simulink model "missile_simulator"  (R2022b)
settings: Solver=VariableStepAuto  StartTime=0.0  StopTime=10  RelTol=1e-3
libraries: vrlib x9
settings Model: Creator=백창인  LastModifiedBy=snow

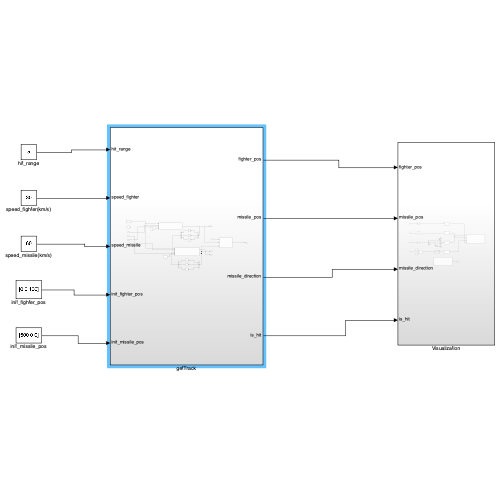
[thumbnail: Simulink's stored preview of the top-level diagram]
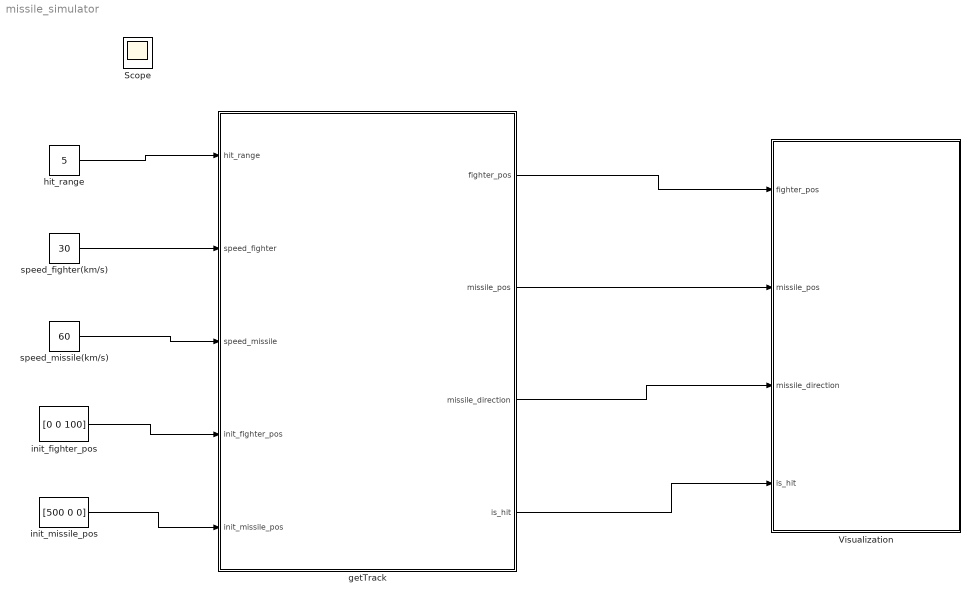
== system missile_simulator ==
  Visualization : Subsystem
  getTrack : Subsystem
  hit_range : Constant  Value=5
  init_fighter_pos : Constant  Value=[0 0 100]
  init_missile_pos : Constant  Value=[500 0 0]
  speed_fighter(km/s) : Constant  Value=30
  speed_missile(km/s) : Constant  Value=60
  Scope : Scope
  wires:
  hit_range/1 -> getTrack/1(hit_range)
  speed_fighter(km/s)/1 -> getTrack/2(speed_fighter)
  speed_missile(km/s)/1 -> getTrack/3(speed_missile)
  init_fighter_pos/1 -> getTrack/4(init_fighter_pos)
  init_missile_pos/1 -> getTrack/5(init_missile_pos)
  getTrack/3(missile_direction) -> Visualization/3(missile_direction)
  getTrack/2(missile_pos) -> Visualization/2(missile_pos)
  getTrack/1(fighter_pos) -> Visualization/1(fighter_pos)
  getTrack/4(is_hit) -> Visualization/4(is_hit)

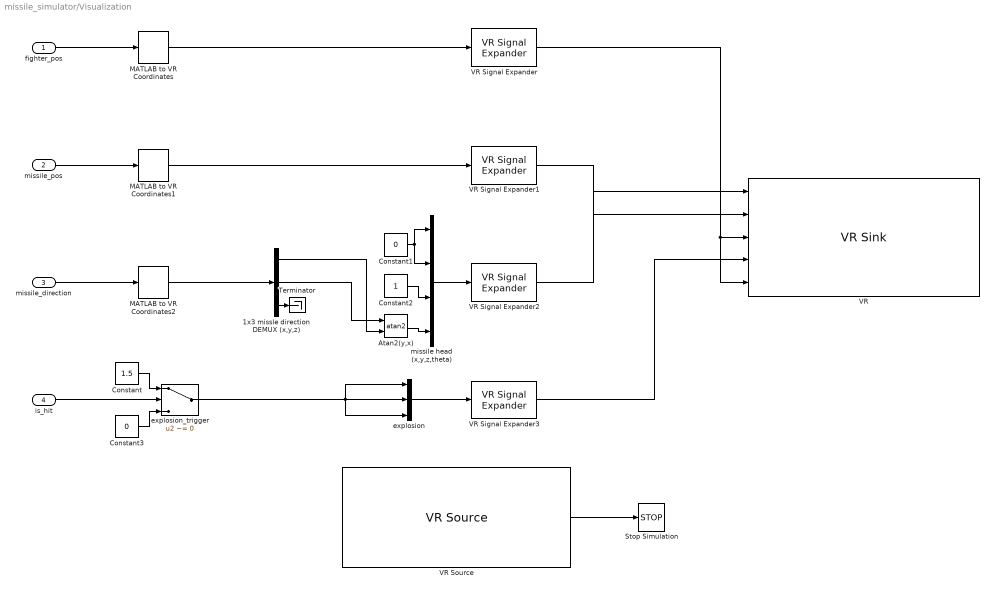
== system missile_simulator/Visualization ==
  fighter_pos : Inport
  missile_pos : Inport  Port=2
  missile_direction : Inport  Port=3
  is_hit : Inport  Port=4
  1x3 missle direction DEMUX (x,y,z) : Demux  Outputs=3
  Atan2(y,x) : Trigonometry  Operator=atan2
  Constant : Constant  Value=1.5
  Constant1 : Constant  Value=0
  Constant2 : Constant
  Constant3 : Constant  Value=0
  MATLAB to VR Coordinates : vrlib/Utilities/MATLAB to VR Coordinates
  MATLAB to VR Coordinates1 : vrlib/Utilities/MATLAB to VR Coordinates
  MATLAB to VR Coordinates2 : vrlib/Utilities/MATLAB to VR Coordinates
  Stop Simulation : Stop
  Terminator : Terminator
  VR : vrlib/VR Sink  InstantiateOnLoad=on  SampleTime=0.01  ViewEnable=on  RemoteChange=off  RemoteView=off  FieldsWritten=missile.rotation.4.1.1.double#missile.translation.3.1.1.double#Fighter.translation.3.1.1.double#explosion.scale.3.1.1.double#explosion.translation.3.1.1.double  WorldFileName=display.x3d  AutoView=on  VideoDimensions=[]  AllowVariableSize=off
  VR Signal Expander : vrlib/VR Signal Expander  outwidth=3  outidx=[1 2 3]
  VR Signal Expander1 : vrlib/VR Signal Expander  outwidth=3  outidx=[1 2 3]
  VR Signal Expander2 : vrlib/VR Signal Expander  outwidth=4  outidx=[1 2 3 4]
  VR Signal Expander3 : vrlib/VR Signal Expander  outwidth=3  outidx=[1 2 3]
  VR Source : vrlib/VR Source  InstantiateOnLoad=on  SampleTime=0.1  ViewEnable=on  RemoteChange=off  RemoteView=off  FieldsRead=explosion.scale.1.3.1.double  WorldFileName=display.x3d  AutoView=off  VideoDimensions=[]  AllowVariableSize=off
  explosion : Mux  Inputs=3
  explosion_trigger : Switch  Criteria=u2 ~= 0  SaturateOnIntegerOverflow=off  InputSameDT=off
  missile head (x,y,z,theta) : Mux
  wires:
  MATLAB to VR Coordinates/1 -> VR Signal Expander/1
  fighter_pos/1 -> MATLAB to VR Coordinates/1
  missile_pos/1 -> MATLAB to VR Coordinates1/1
  MATLAB to VR Coordinates1/1 -> VR Signal Expander1/1
  Constant2/1 -> missile head (x,y,z,theta)/3
  1x3 missle direction DEMUX (x,y,z)/1 -> Atan2(y,x)/2
  1x3 missle direction DEMUX (x,y,z)/2 -> Atan2(y,x)/1
  missile head (x,y,z,theta)/1 -> VR Signal Expander2/1
  Constant1/1 -> missile head (x,y,z,theta)/1, missile head (x,y,z,theta)/2
  Atan2(y,x)/1 -> missile head (x,y,z,theta)/4
  MATLAB to VR Coordinates2/1 -> 1x3 missle direction DEMUX (x,y,z)/1
  missile_direction/1 -> MATLAB to VR Coordinates2/1
  explosion/1 -> VR Signal Expander3/1
  explosion_trigger/1 -> explosion/1, explosion/3, explosion/2
  is_hit/1 -> explosion_trigger/2
  Constant3/1 -> explosion_trigger/3
  Constant/1 -> explosion_trigger/1
  1x3 missle direction DEMUX (x,y,z)/3 -> Terminator/1
  VR Signal Expander2/1 -> VR/1
  VR Signal Expander1/1 -> VR/2
  VR Signal Expander/1 -> VR/3, VR/5
  VR Signal Expander3/1 -> VR/4
  VR Source/1 -> Stop Simulation/1

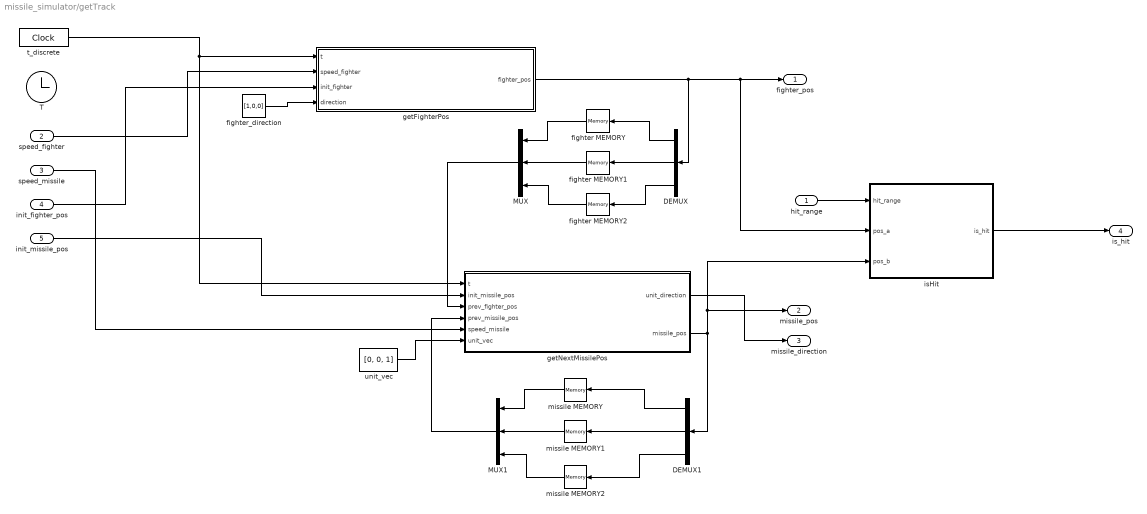
== system missile_simulator/getTrack ==
  hit_range : Inport
  speed_fighter : Inport  Port=2
  speed_missile : Inport  Port=3
  init_fighter_pos : Inport  Port=4
  init_missile_pos : Inport  Port=5
  DEMUX : Demux  Outputs=3
  DEMUX1 : Demux  Outputs=3
  MUX : Mux  Inputs=3
  MUX1 : Mux  Inputs=3
  T : Clock
  fighter MEMORY : Memory  InheritSampleTime=on
  fighter MEMORY1 : Memory  InheritSampleTime=on
  fighter MEMORY2 : Memory  InheritSampleTime=on
  fighter_direction : Constant  Value=[1,0,0]
  getFighterPos : MATLAB Function  TreatAsAtomicUnit=on
  getNextMissilePos : MATLAB Function  TreatAsAtomicUnit=on
  isHit : MATLAB Function  TreatAsAtomicUnit=on
  missile MEMORY : Memory  InheritSampleTime=on
  missile MEMORY1 : Memory  InheritSampleTime=on
  missile MEMORY2 : Memory  InheritSampleTime=on
  t_discrete : DigitalClock  SampleTime=0.001
  unit_vec : Constant  Value=[0, 0, 1]
  fighter_pos : Outport
  missile_pos : Outport  Port=2
  missile_direction : Outport  Port=3
  is_hit : Outport  Port=4
  wires:
  t_discrete/1 -> getNextMissilePos/1(t), getFighterPos/1(t)
  getFighterPos/1(fighter_pos) -> DEMUX/1, isHit/2(pos_a), fighter_pos/1
  speed_fighter/1 -> getFighterPos/2(speed_fighter)
  init_fighter_pos/1 -> getFighterPos/3(init_fighter)
  fighter_direction/1 -> getFighterPos/4(direction)
  getNextMissilePos/2(missile_pos) -> isHit/3(pos_b), missile_pos/1, DEMUX1/1
  init_missile_pos/1 -> getNextMissilePos/2(init_missile_pos)
  speed_missile/1 -> getNextMissilePos/5(speed_missile)
  MUX1/1 -> getNextMissilePos/4(prev_missile_pos)
  MUX/1 -> getNextMissilePos/3(prev_fighter_pos)
  DEMUX/2 -> fighter MEMORY1/1
  DEMUX/1 -> fighter MEMORY/1
  DEMUX/3 -> fighter MEMORY2/1
  fighter MEMORY/1 -> MUX/1
  fighter MEMORY1/1 -> MUX/2
  fighter MEMORY2/1 -> MUX/3
  DEMUX1/1 -> missile MEMORY/1
  DEMUX1/2 -> missile MEMORY1/1
  DEMUX1/3 -> missile MEMORY2/1
  missile MEMORY1/1 -> MUX1/2
  missile MEMORY/1 -> MUX1/1
  missile MEMORY2/1 -> MUX1/3
  isHit/1(is_hit) -> is_hit/1
  hit_range/1 -> isHit/1(hit_range)
  getNextMissilePos/1(unit_direction) -> missile_direction/1
  unit_vec/1 -> getNextMissilePos/6(unit_vec)

== matlab function missile_simulator/getTrack/isHit ==
  data: hit_range input; is_hit output; pos_a input; pos_b input
function is_hit = isHit(hit_range, pos_a, pos_b)
    is_hit = 0;
    distance = norm(pos_a - pos_b);

    if (distance <= hit_range)
        is_hit = 1;
    end
end

== matlab function missile_simulator/getTrack/getFighterPos ==
  data: t input; fighter_pos output; speed_fighter input; init_fighter input; direction input
function fighter_pos = getFighterPos(t,speed_fighter,init_fighter,direction)
    position = init_fighter + t*direction*speed_fighter; %전투기의 위치를 속도와 시간에 따라 재설정
fighter_pos = position;
end

== matlab function missile_simulator/getTrack/getNextMissilePos ==
  data: unit_direction output; t input; init_missile_pos input; prev_fighter_pos input; prev_missile_pos input; missile_pos output; speed_missile input; unit_vec input
function [unit_direction, missile_pos] = getNextMissilePos(t, init_missile_pos, prev_fighter_pos, prev_missile_pos, speed_missile, unit_vec)
% 방향벡터에 미사일 속도를 적용
if (t==0) %초기값
    missile_pos = init_missile_pos;
    unit_direction = unit_vec;
else
    direction = (prev_fighter_pos - prev_missile_pos); %미사일 방향벡터
    unit_direction = (direction)/norm(direction);
    missile_pos = prev_missile_pos + (speed_missile/1000) * unit_direction;
end

end
